simulink library "Storage_Type_1"  (R2016b)
settings: Solver=ode45  StartTime=0.0  StopTime=10.0  RelTol=1e-3  EnableMultiTasking=on
libraries: carnot x6
settings Model: Creator=lena.frank  LastModifiedBy=drhf
settings DataIOCC: LimitDataPoints=on  SaveFormat=Array  SignalLoggingSaveFormat=ModelDataLogs
settings OptimizationCC: ExpressionDepthLimit=2147483647  LifeSpan=inf
settings DebuggingCC: UnderspecifiedInitializationDetection=Classic  MergeDetectMultiDrivingBlocksExec=none  SolverPrmCheckMsg=warning  FcnCallInpInsideContextMsg=warning  StateNameClashWarn=warning  SFUnexpectedBacktrackingDiag=warning  SFNoUnconditionalDefaultTransitionDiag=warning  SFExecutionAtInitializationDiag=none
settings HardwareCC: ProdBitPerPointer=32  ProdBitPerSizeT=32  ProdBitPerPtrDiffT=32  ProdLargestAtomicFloat=None  ProdIntDivRoundTo=Undefined  ProdEndianess=Unspecified  ProdWordSize=32  ProdHWDeviceType=32-bit Generic
settings ModelReferenceCC: PropagateSignalLabelsOutOfModel=off
settings GRTTargetCC: TargetLangStandard=C89/C90 (ANSI)  GeneratePreprocessorConditionals=Disable all  CombineOutputUpdateFcns=off  GRTInterface=on
settings ConfigComp: CovMetricSettings=dw  CovHtmlReporting=on  CovSaveCumulativeToWorkspaceVar=on  CovSaveSingleToWorkspaceVar=on  CovExternalEMLEnable=off

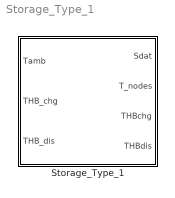
== system Storage_Type_1 ==
  Storage_Type_1 : Subsystem  mask(Multiport Storage){uloss=1, ubot=1, utop=1, cond=1, volume=0.5, dia=0.6, pos=standing cylinder, h_in_chg=1, h_out_chg=0, pipe1dia=0.03, h_in=0, h_out=1, pipe2dia=0.03, t0=[10:5:55], nodes=10, mpoints=10}
      mask prompts: uloss "Heat transfer coefficient to ambient [W/m²K]"; ubot "Heat transfer coefficient to ambient bottom [W/m²K]"; utop "Heat transfer coefficient to ambient top [W/m²K]"; cond "effective thermal conductivity [W/mK]"; volume "Volume [m³]"; dia "Diameter [m]"; pos "Position"; h_in_chg "relative height of inlet, range = 0 (bottom) to 1 (top)"; h_out_chg "relative height of outlet, range = 0 (bottom) to 1 (top)"; pipe1dia "Diameter of pipe in m"; h_in "relative height of inlet, range = 0 (bottom) to 1 (top)"; h_out "relative height of outlet, range = 0 (bottom) to 1 (top)"; pipe2dia "Diameter of pipe in m"; t0 "Initial temperature (vector or scalar) in °C"; nodes "Number of nodes"; mpoints "Number of measurement points"
      mask help:
      | The volmue of the cylindrical storage is divided in a number "nodes" of horizontal slices (1xN-node model). For each node the energy balance equation is solved.
      | Parameters from underlying sub-masks are promoted by top mask.
      mask init:
      | [standing, dh, height, mpts, tini] ...
      |     = CarnotCallbacks_StorageTypeN(pos, volume, dia, nodes, mpoints, t0);
      mask Help: web(fullfile(path_carnot('help'),'Storage_Type_N.html'),'-helpbrowser')
      mask TypeOptions uloss: sfun_storageTnodes/uloss
      mask TypeOptions ubot: sfun_storageTnodes/ubot
      mask TypeOptions utop: sfun_storageTnodes/utop
      mask TypeOptions cond: sfun_storageTnodes/cond
      mask TypeOptions volume: sfun_storageTnodes/volume | CreateSdat/volume
      mask TypeOptions dia: sfun_storageTnodes/dia
      mask TypeOptions pos: lying cylinder | standing cylinder
      mask TypeOptions h_in_chg: pipe_charge/h_in
      mask TypeOptions h_out_chg: pipe_charge/h_out
      mask TypeOptions pipe1dia: pipe_charge/dia
      mask TypeOptions h_in: pipe_discharge/h_in
      mask TypeOptions h_out: pipe_discharge/h_out
      mask TypeOptions pipe2dia: pipe_discharge/dia
      mask TypeOptions nodes: sfun_storageTnodes/nodes | pipe_charge/nodes | pipe_discharge/nodes | select_T/InputPortWidth
      mask Display: plot(10,10,90,100,[40,40,45,55,60,60,55,45,40],[84,36,30,30,36,84,90,90,84],[40,35],[77,77],[64,60],[77,77],[40,35],[42,42],[64,60],[42,42])

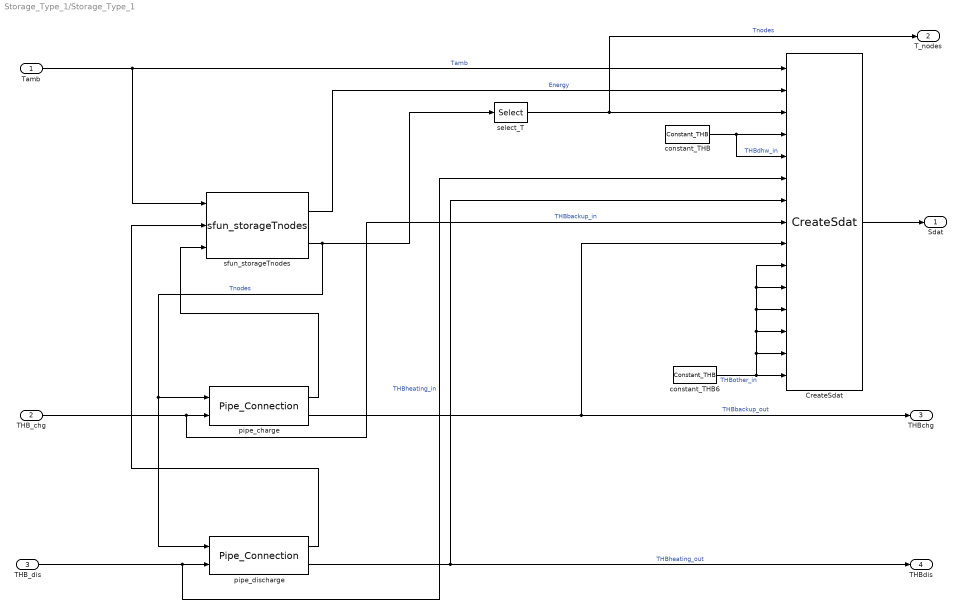
== system Storage_Type_1/Storage_Type_1 ==
  Tamb : Inport
  THB_chg : Inport  Port=2
  THB_dis : Inport  Port=3
  CreateSdat : carnot/Basic/Thermal_Models/CreateSdat  volume=volume  stgtype=1
  constant_THB : carnot/Source/Simple/Constant_THB  t=20  mdot=0  p=1e5  mID=No Pressure Drop  fluid=Water  mix=0  mix2=0  mix3=0  dia=0.02  hgt=0
  constant_THB6 : carnot/Source/Simple/Constant_THB  t=20  mdot=0  p=1e5  mID=No Pressure Drop  fluid=Water  mix=0  mix2=0  mix3=0  dia=0.02  hgt=0
  pipe_charge : carnot/Storage/Thermal/Storage_Ports/Pipe_Connection  h_in=h_in_chg  h_out=h_out_chg  hgt=height  dia=pipe1dia  nodes=nodes
  pipe_discharge : carnot/Storage/Thermal/Storage_Ports/Pipe_Connection  h_in=h_in  h_out=h_out  hgt=height  dia=pipe2dia  nodes=nodes
  select_T : Selector  InputPortWidth=nodes  IndexOptions=Index vector (dialog)  Indices=mpts  OutputSizes=1
  sfun_storageTnodes : carnot/Basic/Thermal_Models/sfun_storageTnodes  uloss=uloss  ubot=ubot  utop=utop  cond=cond  volume=volume  dia=dia  standing=standing cylinder  tini=tini  nodes=nodes  nconnect=2  elimthermocline=2  condinvtc=1e5
  Sdat : Outport
  T_nodes : Outport  Port=2
  THBchg : Outport  Port=3
  THBdis : Outport  Port=4
  wires:
  pipe_charge/1 -> sfun_storageTnodes/3
  pipe_charge/2 -> CreateSdat/9, THBchg/1  "THBbackup_out"
  THB_chg/1 -> CreateSdat/8, pipe_charge/2  "THBbackup_in"
  constant_THB6/1 -> CreateSdat/15, CreateSdat/14, CreateSdat/13, CreateSdat/12, CreateSdat/11, CreateSdat/10  "THBother_in"
  CreateSdat/1 -> Sdat/1
  constant_THB/1 -> CreateSdat/4, CreateSdat/5  "THBdhw_in"
  sfun_storageTnodes/2 -> select_T/1, pipe_discharge/1, pipe_charge/1  "Tnodes"
  sfun_storageTnodes/1 -> CreateSdat/2  "Energy"
  select_T/1 -> CreateSdat/3, T_nodes/1  "Tnodes"
  pipe_discharge/1 -> sfun_storageTnodes/2
  pipe_discharge/2 -> CreateSdat/7, THBdis/1  "THBheating_out"
  THB_dis/1 -> CreateSdat/6, pipe_discharge/2  "THBheating_in"
  Tamb/1 -> CreateSdat/1, sfun_storageTnodes/1  "Tamb"
